simulink model "My_Nonlinear_with_controller_draft"  (R2021b)
settings: Solver=VariableStepAuto  StartTime=0.0  StopTime=simTime  RelTol=1e-3
undefined symbols (not defined in the file): att_Kd, att_Ki, att_Kp, b, D, g, k, L, m, MoI, omega, p, p_dot, posZ_Kd, posZ_Ki, posZ_Kp, posZ_N, Theta, TorV
libraries: slpidlib x8
settings Model: Creator=tanzc  LastModifiedBy=tanzc

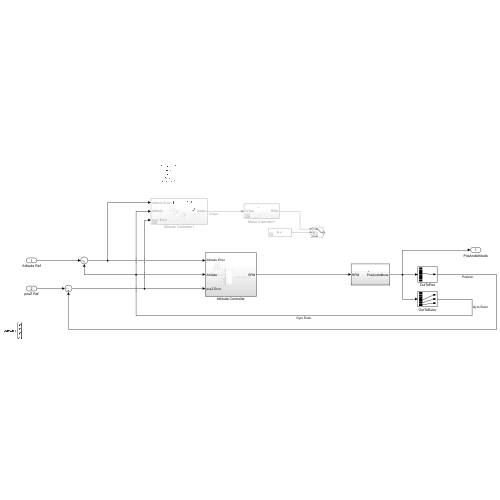
[thumbnail: Simulink's stored preview of the top-level diagram]
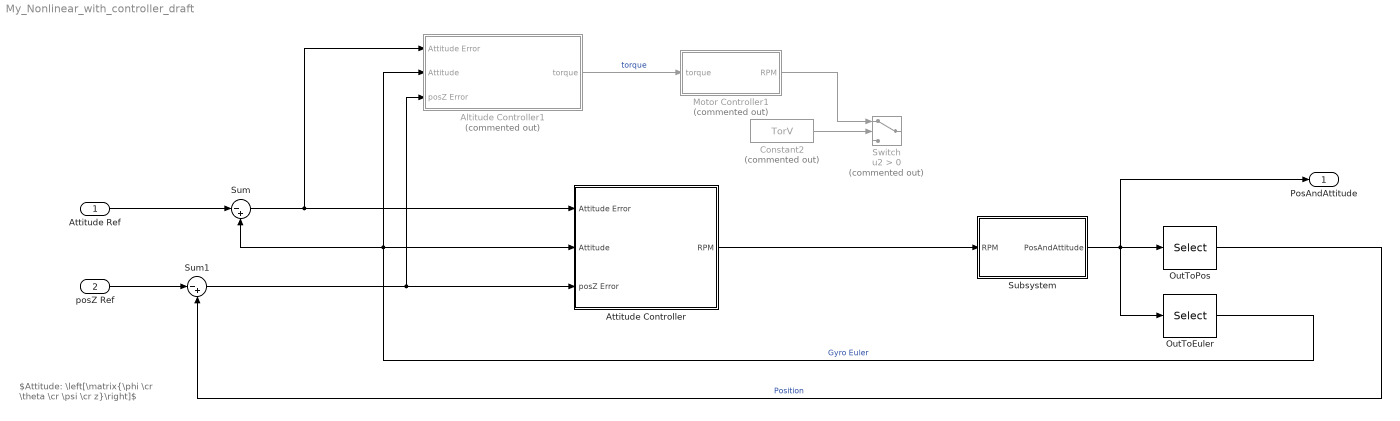
== system My_Nonlinear_with_controller_draft ==
  note: $Attitude: \left[\matrix{\phi \cr \theta \cr \psi \cr z}\right]$
  Attitude Ref : Inport  PortDimensions=3
  posZ Ref : Inport  Port=2  PortDimensions=1
  Altitude Controller1 : Subsystem  Commented=on
  Attitude Controller : Subsystem
  Constant2 : Constant  Commented=on  Value=TorV
  Motor Controller1 : Subsystem  Commented=on
  OutToEuler : Selector  InputPortWidth=6  IndexOptions=Index vector (dialog)  Indices=[4 5 6]  OutputSizes=1
  OutToPos : Selector  InputPortWidth=6  IndexOptions=Index vector (dialog)  Indices=[3]  OutputSizes=1
  Subsystem : Subsystem
  Sum : Sum  Inputs=|-+
  Sum1 : Sum  Inputs=|-+
  Switch : Switch  Commented=on  Criteria=u2 > Threshold
  PosAndAttitude : Outport
  wires:
  Subsystem/1(PosAndAttitude) -> PosAndAttitude/1, OutToEuler/1, OutToPos/1
  OutToPos/1 -> Sum1/2  "Position"
  OutToEuler/1 -> Altitude Controller1/2(Attitude), Attitude Controller/2(Attitude), Sum/2  "Gyro Euler"
  Sum/1 -> Altitude Controller1/1(Attitude Error), Attitude Controller/1(Attitude Error)
  Attitude Ref/1 -> Sum/1
  posZ Ref/1 -> Sum1/1
  Sum1/1 -> Altitude Controller1/3(posZ Error), Attitude Controller/3(posZ Error)
  Motor Controller1/1(RPM) -> Switch/1
  Constant2/1 -> Switch/2
  Altitude Controller1/1(torque) -> Motor Controller1/1(torque)  "torque"
  Attitude Controller/1(RPM) -> Subsystem/1(RPM)

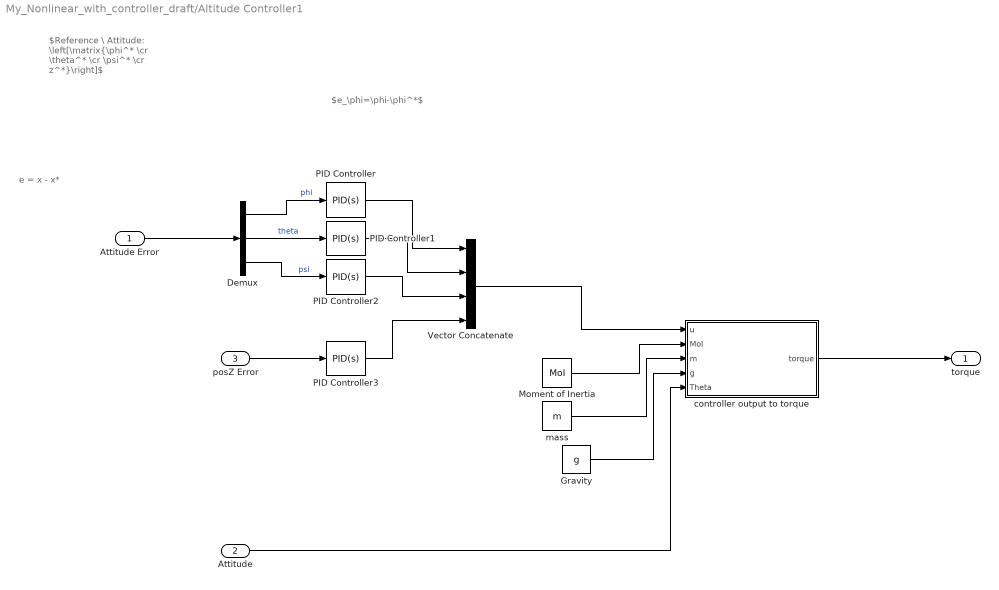
== system My_Nonlinear_with_controller_draft/Altitude Controller1 ==
  note: e = x - x*
  note: $e_\phi=\phi-\phi^*$
  note: $Reference \ Attitude: \left[\matrix{\phi^* \cr \theta^* \cr \psi^* \cr z^*}\right]$
  Attitude Error : Inport
  Attitude : Inport  Port=2
  posZ Error : Inport  Port=3
  Demux : Demux  Outputs=3
  Gravity : Constant  Value=g  VectorParams1D=off
  Moment of Inertia : Constant  Value=MoI  VectorParams1D=off
  PID Controller : slpidlib/PID Controller  Controller=PID  Form=Parallel  TimeDomain=Continuous-time  UseExternalTs=off  SampleTime=-1  IntegratorMethod=Forward Euler  FilterMethod=Forward Euler  ControllerParametersSource=internal  P=att_Kp  I=att_Ki  D=att_Kd  UseFilter=on  N=100  TunerSelectOption=Transfer Function Based (PID Tuner App)  InitialConditionSource=internal  InitialConditionForIntegrator=0  InitialConditionForFilter=0  DifferentiatorICPrevScaledInput=0  ExternalReset=none  TrackingMode=off  Kt=1  LimitOutput=off  SatLimitsSource=internal  UpperSaturationLimit=inf  LowerSaturationLimit=-inf  LinearizeAsGain=on  AntiWindupMode=none  Kb=1  POutMin=[]  POutMax=[]  IOutMin=[]  IOutMax=[]  DOutMin=[]  DOutMax=[]  NOutMin=[]  NOutMax=[]  SumOutMin=[]  SumOutMax=[]  SaturationOutMin=[]  SaturationOutMax=[]  PParamMin=[]  PParamMax=[]  IParamMin=[]  IParamMax=[]  DParamMin=[]  DParamMax=[]  NParamMin=[]  NParamMax=[]  KbParamMin=[]  KbParamMax=[]  KtParamMin=[]  KtParamMax=[]  KbOutMin=[]  KbOutMax=[]  KtOutMin=[]  KtOutMax=[]  IntegratorOutMin=[]  IntegratorOutMax=[]  FilterOutMin=[]  FilterOutMax=[]  SumI1OutMin=[]  SumI1OutMax=[]  SumI2OutMin=[]  SumI2OutMax=[]  SumI3OutMin=[]  SumI3OutMax=[]  SumI4OutMin=[]  SumI4OutMax=[]  SumDOutMin=[]  SumDOutMax=[]  DifferentiatorOutMin=[]  DifferentiatorOutMax=[]  FilterDiffOutCoefMin=[]  FilterDiffOutCoefMax=[]  ReciprocalOutMin=[]  ReciprocalOutMax=[]  SumDenOutMin=[]  SumDenOutMax=[]  SumNumOutMin=[]  SumNumOutMax=[]  DivideOutMin=[]  DivideOutMax=[]  UdiffTsProdOutMin=[]  UdiffTsProdOutMax=[]  NTsProdOutMin=[]  NTsProdOutMax=[]  UintegralTsProdOutMin=[]  UintegralTsProdOutMax=[]  UngainTsProdOutMin=[]  UngainTsProdOutMax=[]  IntegratorContinuousStateAttributes=''  IntegratorStateMustResolveToSignalObject=off  IntegratorRTWStateStorageClass=Auto  FilterContinuousStateAttributes=''  FilterStateMustResolveToSignalObject=off  FilterRTWStateStorageClass=Auto  ParallelPVariant=InternalParameters  IdealPVariant=Disabled  IVariant=InternalParameters  DVariant=InternalParameters  IntegratorVariant=Continuous  SatVariant=Disabled  AWVariant=Passthrough  PCopyVariant=Disabled  TRVariant=Disabled  FdbkBlocksVariant=Forward  IdealPFdbkVariant=Disabled  SatFdbkVariant=Disabled  DerivativeFilterVariant=ContFilter  NVariant=InternalParameters  NCopyVariant=Disabled  FilterICVariant=InternalICsFilter  IntegratorICVariant=InternalICs  ExternalResetVariant=Disabled  TRSumVariant=Passthrough  SumFdbkVariant=Disabled  SumVariant=Sum_PID  TsampFilterVariant=InternalTs  TsampNgainVariant=Passthrough  TsampIntegralVariant=Passthrough  ExternalSaturationOutDataTypeStr=Inherit: Same as second input
  PID Controller1 : slpidlib/PID Controller  Controller=PID  Form=Parallel  TimeDomain=Continuous-time  UseExternalTs=off  SampleTime=-1  IntegratorMethod=Forward Euler  FilterMethod=Forward Euler  ControllerParametersSource=internal  P=att_Kp  I=att_Ki  D=att_Kd  UseFilter=on  N=100  TunerSelectOption=Transfer Function Based (PID Tuner App)  InitialConditionSource=internal  InitialConditionForIntegrator=0  InitialConditionForFilter=0  DifferentiatorICPrevScaledInput=0  ExternalReset=none  TrackingMode=off  Kt=1  LimitOutput=off  SatLimitsSource=internal  UpperSaturationLimit=inf  LowerSaturationLimit=-inf  LinearizeAsGain=on  AntiWindupMode=none  Kb=1  POutMin=[]  POutMax=[]  IOutMin=[]  IOutMax=[]  DOutMin=[]  DOutMax=[]  NOutMin=[]  NOutMax=[]  SumOutMin=[]  SumOutMax=[]  SaturationOutMin=[]  SaturationOutMax=[]  PParamMin=[]  PParamMax=[]  IParamMin=[]  IParamMax=[]  DParamMin=[]  DParamMax=[]  NParamMin=[]  NParamMax=[]  KbParamMin=[]  KbParamMax=[]  KtParamMin=[]  KtParamMax=[]  KbOutMin=[]  KbOutMax=[]  KtOutMin=[]  KtOutMax=[]  IntegratorOutMin=[]  IntegratorOutMax=[]  FilterOutMin=[]  FilterOutMax=[]  SumI1OutMin=[]  SumI1OutMax=[]  SumI2OutMin=[]  SumI2OutMax=[]  SumI3OutMin=[]  SumI3OutMax=[]  SumI4OutMin=[]  SumI4OutMax=[]  SumDOutMin=[]  SumDOutMax=[]  DifferentiatorOutMin=[]  DifferentiatorOutMax=[]  FilterDiffOutCoefMin=[]  FilterDiffOutCoefMax=[]  ReciprocalOutMin=[]  ReciprocalOutMax=[]  SumDenOutMin=[]  SumDenOutMax=[]  SumNumOutMin=[]  SumNumOutMax=[]  DivideOutMin=[]  DivideOutMax=[]  UdiffTsProdOutMin=[]  UdiffTsProdOutMax=[]  NTsProdOutMin=[]  NTsProdOutMax=[]  UintegralTsProdOutMin=[]  UintegralTsProdOutMax=[]  UngainTsProdOutMin=[]  UngainTsProdOutMax=[]  IntegratorContinuousStateAttributes=''  IntegratorStateMustResolveToSignalObject=off  IntegratorRTWStateStorageClass=Auto  FilterContinuousStateAttributes=''  FilterStateMustResolveToSignalObject=off  FilterRTWStateStorageClass=Auto  ParallelPVariant=InternalParameters  IdealPVariant=Disabled  IVariant=InternalParameters  DVariant=InternalParameters  IntegratorVariant=Continuous  SatVariant=Disabled  AWVariant=Passthrough  PCopyVariant=Disabled  TRVariant=Disabled  FdbkBlocksVariant=Forward  IdealPFdbkVariant=Disabled  SatFdbkVariant=Disabled  DerivativeFilterVariant=ContFilter  NVariant=InternalParameters  NCopyVariant=Disabled  FilterICVariant=InternalICsFilter  IntegratorICVariant=InternalICs  ExternalResetVariant=Disabled  TRSumVariant=Passthrough  SumFdbkVariant=Disabled  SumVariant=Sum_PID  TsampFilterVariant=InternalTs  TsampNgainVariant=Passthrough  TsampIntegralVariant=Passthrough  ExternalSaturationOutDataTypeStr=Inherit: Same as second input
  PID Controller2 : slpidlib/PID Controller  Controller=PID  Form=Parallel  TimeDomain=Continuous-time  UseExternalTs=off  SampleTime=-1  IntegratorMethod=Forward Euler  FilterMethod=Forward Euler  ControllerParametersSource=internal  P=att_Kp  I=att_Ki  D=att_Kd  UseFilter=on  N=100  TunerSelectOption=Transfer Function Based (PID Tuner App)  InitialConditionSource=internal  InitialConditionForIntegrator=0  InitialConditionForFilter=0  DifferentiatorICPrevScaledInput=0  ExternalReset=none  TrackingMode=off  Kt=1  LimitOutput=off  SatLimitsSource=internal  UpperSaturationLimit=inf  LowerSaturationLimit=-inf  LinearizeAsGain=on  AntiWindupMode=none  Kb=1  POutMin=[]  POutMax=[]  IOutMin=[]  IOutMax=[]  DOutMin=[]  DOutMax=[]  NOutMin=[]  NOutMax=[]  SumOutMin=[]  SumOutMax=[]  SaturationOutMin=[]  SaturationOutMax=[]  PParamMin=[]  PParamMax=[]  IParamMin=[]  IParamMax=[]  DParamMin=[]  DParamMax=[]  NParamMin=[]  NParamMax=[]  KbParamMin=[]  KbParamMax=[]  KtParamMin=[]  KtParamMax=[]  KbOutMin=[]  KbOutMax=[]  KtOutMin=[]  KtOutMax=[]  IntegratorOutMin=[]  IntegratorOutMax=[]  FilterOutMin=[]  FilterOutMax=[]  SumI1OutMin=[]  SumI1OutMax=[]  SumI2OutMin=[]  SumI2OutMax=[]  SumI3OutMin=[]  SumI3OutMax=[]  SumI4OutMin=[]  SumI4OutMax=[]  SumDOutMin=[]  SumDOutMax=[]  DifferentiatorOutMin=[]  DifferentiatorOutMax=[]  FilterDiffOutCoefMin=[]  FilterDiffOutCoefMax=[]  ReciprocalOutMin=[]  ReciprocalOutMax=[]  SumDenOutMin=[]  SumDenOutMax=[]  SumNumOutMin=[]  SumNumOutMax=[]  DivideOutMin=[]  DivideOutMax=[]  UdiffTsProdOutMin=[]  UdiffTsProdOutMax=[]  NTsProdOutMin=[]  NTsProdOutMax=[]  UintegralTsProdOutMin=[]  UintegralTsProdOutMax=[]  UngainTsProdOutMin=[]  UngainTsProdOutMax=[]  IntegratorContinuousStateAttributes=''  IntegratorStateMustResolveToSignalObject=off  IntegratorRTWStateStorageClass=Auto  FilterContinuousStateAttributes=''  FilterStateMustResolveToSignalObject=off  FilterRTWStateStorageClass=Auto  ParallelPVariant=InternalParameters  IdealPVariant=Disabled  IVariant=InternalParameters  DVariant=InternalParameters  IntegratorVariant=Continuous  SatVariant=Disabled  AWVariant=Passthrough  PCopyVariant=Disabled  TRVariant=Disabled  FdbkBlocksVariant=Forward  IdealPFdbkVariant=Disabled  SatFdbkVariant=Disabled  DerivativeFilterVariant=ContFilter  NVariant=InternalParameters  NCopyVariant=Disabled  FilterICVariant=InternalICsFilter  IntegratorICVariant=InternalICs  ExternalResetVariant=Disabled  TRSumVariant=Passthrough  SumFdbkVariant=Disabled  SumVariant=Sum_PID  TsampFilterVariant=InternalTs  TsampNgainVariant=Passthrough  TsampIntegralVariant=Passthrough  ExternalSaturationOutDataTypeStr=Inherit: Same as second input
  PID Controller3 : slpidlib/PID Controller  Controller=PID  Form=Parallel  TimeDomain=Continuous-time  UseExternalTs=off  SampleTime=-1  IntegratorMethod=Forward Euler  FilterMethod=Forward Euler  ControllerParametersSource=internal  P=posZ_Kp  I=posZ_Ki  D=posZ_Kd  UseFilter=on  N=100  TunerSelectOption=Transfer Function Based (PID Tuner App)  InitialConditionSource=internal  InitialConditionForIntegrator=0  InitialConditionForFilter=0  DifferentiatorICPrevScaledInput=0  ExternalReset=none  TrackingMode=off  Kt=1  LimitOutput=off  SatLimitsSource=internal  UpperSaturationLimit=inf  LowerSaturationLimit=-inf  LinearizeAsGain=on  AntiWindupMode=none  Kb=1  POutMin=[]  POutMax=[]  IOutMin=[]  IOutMax=[]  DOutMin=[]  DOutMax=[]  NOutMin=[]  NOutMax=[]  SumOutMin=[]  SumOutMax=[]  SaturationOutMin=[]  SaturationOutMax=[]  PParamMin=[]  PParamMax=[]  IParamMin=[]  IParamMax=[]  DParamMin=[]  DParamMax=[]  NParamMin=[]  NParamMax=[]  KbParamMin=[]  KbParamMax=[]  KtParamMin=[]  KtParamMax=[]  KbOutMin=[]  KbOutMax=[]  KtOutMin=[]  KtOutMax=[]  IntegratorOutMin=[]  IntegratorOutMax=[]  FilterOutMin=[]  FilterOutMax=[]  SumI1OutMin=[]  SumI1OutMax=[]  SumI2OutMin=[]  SumI2OutMax=[]  SumI3OutMin=[]  SumI3OutMax=[]  SumI4OutMin=[]  SumI4OutMax=[]  SumDOutMin=[]  SumDOutMax=[]  DifferentiatorOutMin=[]  DifferentiatorOutMax=[]  FilterDiffOutCoefMin=[]  FilterDiffOutCoefMax=[]  ReciprocalOutMin=[]  ReciprocalOutMax=[]  SumDenOutMin=[]  SumDenOutMax=[]  SumNumOutMin=[]  SumNumOutMax=[]  DivideOutMin=[]  DivideOutMax=[]  UdiffTsProdOutMin=[]  UdiffTsProdOutMax=[]  NTsProdOutMin=[]  NTsProdOutMax=[]  UintegralTsProdOutMin=[]  UintegralTsProdOutMax=[]  UngainTsProdOutMin=[]  UngainTsProdOutMax=[]  IntegratorContinuousStateAttributes=''  IntegratorStateMustResolveToSignalObject=off  IntegratorRTWStateStorageClass=Auto  FilterContinuousStateAttributes=''  FilterStateMustResolveToSignalObject=off  FilterRTWStateStorageClass=Auto  ParallelPVariant=InternalParameters  IdealPVariant=Disabled  IVariant=InternalParameters  DVariant=InternalParameters  IntegratorVariant=Continuous  SatVariant=Disabled  AWVariant=Passthrough  PCopyVariant=Disabled  TRVariant=Disabled  FdbkBlocksVariant=Forward  IdealPFdbkVariant=Disabled  SatFdbkVariant=Disabled  DerivativeFilterVariant=ContFilter  NVariant=InternalParameters  NCopyVariant=Disabled  FilterICVariant=InternalICsFilter  IntegratorICVariant=InternalICs  ExternalResetVariant=Disabled  TRSumVariant=Passthrough  SumFdbkVariant=Disabled  SumVariant=Sum_PID  TsampFilterVariant=InternalTs  TsampNgainVariant=Passthrough  TsampIntegralVariant=Passthrough  ExternalSaturationOutDataTypeStr=Inherit: Same as second input
  Vector Concatenate : Concatenate  NumInputs=4
  controller output to torque : MATLAB Function  TreatAsAtomicUnit=on
  mass : Constant  Value=m
  torque : Outport
  wires:
  Attitude Error/1 -> Demux/1
  Attitude/1 -> controller output to torque/5(Theta)
  Vector Concatenate/1 -> controller output to torque/1(u)
  Moment of Inertia/1 -> controller output to torque/2(MoI)
  mass/1 -> controller output to torque/3(m)
  Gravity/1 -> controller output to torque/4(g)
  controller output to torque/1(torque) -> torque/1
  Demux/1 -> PID Controller/1  "phi"
  Demux/2 -> PID Controller1/1  "theta"
  Demux/3 -> PID Controller2/1  "psi"
  posZ Error/1 -> PID Controller3/1
  PID Controller/1 -> Vector Concatenate/1
  PID Controller1/1 -> Vector Concatenate/2
  PID Controller2/1 -> Vector Concatenate/3
  PID Controller3/1 -> Vector Concatenate/4

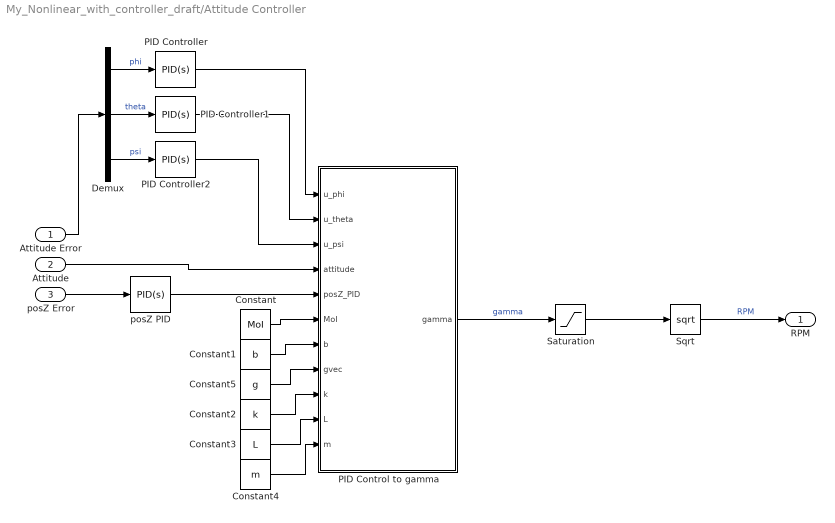
== system My_Nonlinear_with_controller_draft/Attitude Controller ==
  Attitude Error : Inport  PortDimensions=3
  Attitude : Inport  Port=2  PortDimensions=3
  posZ Error : Inport  Port=3
  Constant : Constant  Value=MoI
  Constant1 : Constant  Value=b
  Constant2 : Constant  Value=k
  Constant3 : Constant  Value=L
  Constant4 : Constant  Value=m
  Constant5 : Constant  Value=g
  Demux : Demux  Outputs=3
  PID Control to gamma : MATLAB Function  TreatAsAtomicUnit=on
  PID Controller : slpidlib/PID Controller  Priority=1  Controller=PID  Form=Parallel  TimeDomain=Continuous-time  UseExternalTs=off  SampleTime=-1  IntegratorMethod=Forward Euler  FilterMethod=Forward Euler  ControllerParametersSource=internal  P=att_Kp  I=att_Ki  D=att_Kd  UseFilter=on  N=1142.8279760416  TunerSelectOption=Transfer Function Based (PID Tuner App)  InitialConditionSource=internal  InitialConditionForIntegrator=0  InitialConditionForFilter=0  DifferentiatorICPrevScaledInput=0  ExternalReset=none  TrackingMode=off  Kt=1  LimitOutput=off  SatLimitsSource=internal  UpperSaturationLimit=inf  LowerSaturationLimit=-inf  LinearizeAsGain=on  AntiWindupMode=none  Kb=1  POutMin=[]  POutMax=[]  IOutMin=[]  IOutMax=[]  DOutMin=[]  DOutMax=[]  NOutMin=[]  NOutMax=[]  SumOutMin=[]  SumOutMax=[]  SaturationOutMin=[]  SaturationOutMax=[]  PParamMin=[]  PParamMax=[]  IParamMin=[]  IParamMax=[]  DParamMin=[]  DParamMax=[]  NParamMin=[]  NParamMax=[]  KbParamMin=[]  KbParamMax=[]  KtParamMin=[]  KtParamMax=[]  KbOutMin=[]  KbOutMax=[]  KtOutMin=[]  KtOutMax=[]  IntegratorOutMin=[]  IntegratorOutMax=[]  FilterOutMin=[]  FilterOutMax=[]  SumI1OutMin=[]  SumI1OutMax=[]  SumI2OutMin=[]  SumI2OutMax=[]  SumI3OutMin=[]  SumI3OutMax=[]  SumI4OutMin=[]  SumI4OutMax=[]  SumDOutMin=[]  SumDOutMax=[]  DifferentiatorOutMin=[]  DifferentiatorOutMax=[]  FilterDiffOutCoefMin=[]  FilterDiffOutCoefMax=[]  ReciprocalOutMin=[]  ReciprocalOutMax=[]  SumDenOutMin=[]  SumDenOutMax=[]  SumNumOutMin=[]  SumNumOutMax=[]  DivideOutMin=[]  DivideOutMax=[]  UdiffTsProdOutMin=[]  UdiffTsProdOutMax=[]  NTsProdOutMin=[]  NTsProdOutMax=[]  UintegralTsProdOutMin=[]  UintegralTsProdOutMax=[]  UngainTsProdOutMin=[]  UngainTsProdOutMax=[]  IntegratorContinuousStateAttributes=''  IntegratorStateMustResolveToSignalObject=off  IntegratorRTWStateStorageClass=Auto  FilterContinuousStateAttributes=''  FilterStateMustResolveToSignalObject=off  FilterRTWStateStorageClass=Auto  ParallelPVariant=InternalParameters  IdealPVariant=Disabled  IVariant=InternalParameters  DVariant=InternalParameters  IntegratorVariant=Continuous  SatVariant=Disabled  AWVariant=Passthrough  PCopyVariant=Disabled  TRVariant=Disabled  FdbkBlocksVariant=Forward  IdealPFdbkVariant=Disabled  SatFdbkVariant=Disabled  DerivativeFilterVariant=ContFilter  NVariant=InternalParameters  NCopyVariant=Disabled  FilterICVariant=InternalICsFilter  IntegratorICVariant=InternalICs  ExternalResetVariant=Disabled  TRSumVariant=Passthrough  SumFdbkVariant=Disabled  SumVariant=Sum_PID  TsampFilterVariant=InternalTs  TsampNgainVariant=Passthrough  TsampIntegralVariant=Passthrough  ExternalSaturationOutDataTypeStr=Inherit: Same as second input
  PID Controller1 : slpidlib/PID Controller  Priority=2  Controller=PID  Form=Parallel  TimeDomain=Continuous-time  UseExternalTs=off  SampleTime=-1  IntegratorMethod=Forward Euler  FilterMethod=Forward Euler  ControllerParametersSource=internal  P=att_Kp  I=att_Ki  D=att_Kd  UseFilter=on  N=100  TunerSelectOption=Transfer Function Based (PID Tuner App)  InitialConditionSource=internal  InitialConditionForIntegrator=0  InitialConditionForFilter=0  DifferentiatorICPrevScaledInput=0  ExternalReset=none  TrackingMode=off  Kt=1  LimitOutput=off  SatLimitsSource=internal  UpperSaturationLimit=inf  LowerSaturationLimit=-inf  LinearizeAsGain=on  AntiWindupMode=none  Kb=1  POutMin=[]  POutMax=[]  IOutMin=[]  IOutMax=[]  DOutMin=[]  DOutMax=[]  NOutMin=[]  NOutMax=[]  SumOutMin=[]  SumOutMax=[]  SaturationOutMin=[]  SaturationOutMax=[]  PParamMin=[]  PParamMax=[]  IParamMin=[]  IParamMax=[]  DParamMin=[]  DParamMax=[]  NParamMin=[]  NParamMax=[]  KbParamMin=[]  KbParamMax=[]  KtParamMin=[]  KtParamMax=[]  KbOutMin=[]  KbOutMax=[]  KtOutMin=[]  KtOutMax=[]  IntegratorOutMin=[]  IntegratorOutMax=[]  FilterOutMin=[]  FilterOutMax=[]  SumI1OutMin=[]  SumI1OutMax=[]  SumI2OutMin=[]  SumI2OutMax=[]  SumI3OutMin=[]  SumI3OutMax=[]  SumI4OutMin=[]  SumI4OutMax=[]  SumDOutMin=[]  SumDOutMax=[]  DifferentiatorOutMin=[]  DifferentiatorOutMax=[]  FilterDiffOutCoefMin=[]  FilterDiffOutCoefMax=[]  ReciprocalOutMin=[]  ReciprocalOutMax=[]  SumDenOutMin=[]  SumDenOutMax=[]  SumNumOutMin=[]  SumNumOutMax=[]  DivideOutMin=[]  DivideOutMax=[]  UdiffTsProdOutMin=[]  UdiffTsProdOutMax=[]  NTsProdOutMin=[]  NTsProdOutMax=[]  UintegralTsProdOutMin=[]  UintegralTsProdOutMax=[]  UngainTsProdOutMin=[]  UngainTsProdOutMax=[]  IntegratorContinuousStateAttributes=''  IntegratorStateMustResolveToSignalObject=off  IntegratorRTWStateStorageClass=Auto  FilterContinuousStateAttributes=''  FilterStateMustResolveToSignalObject=off  FilterRTWStateStorageClass=Auto  ParallelPVariant=InternalParameters  IdealPVariant=Disabled  IVariant=InternalParameters  DVariant=InternalParameters  IntegratorVariant=Continuous  SatVariant=Disabled  AWVariant=Passthrough  PCopyVariant=Disabled  TRVariant=Disabled  FdbkBlocksVariant=Forward  IdealPFdbkVariant=Disabled  SatFdbkVariant=Disabled  DerivativeFilterVariant=ContFilter  NVariant=InternalParameters  NCopyVariant=Disabled  FilterICVariant=InternalICsFilter  IntegratorICVariant=InternalICs  ExternalResetVariant=Disabled  TRSumVariant=Passthrough  SumFdbkVariant=Disabled  SumVariant=Sum_PID  TsampFilterVariant=InternalTs  TsampNgainVariant=Passthrough  TsampIntegralVariant=Passthrough  ExternalSaturationOutDataTypeStr=Inherit: Same as second input
  PID Controller2 : slpidlib/PID Controller  Priority=3  Controller=PID  Form=Parallel  TimeDomain=Continuous-time  UseExternalTs=off  SampleTime=-1  IntegratorMethod=Forward Euler  FilterMethod=Forward Euler  ControllerParametersSource=internal  P=att_Kp  I=att_Ki  D=att_Kd  UseFilter=on  N=100  TunerSelectOption=Transfer Function Based (PID Tuner App)  InitialConditionSource=internal  InitialConditionForIntegrator=0  InitialConditionForFilter=0  DifferentiatorICPrevScaledInput=0  ExternalReset=none  TrackingMode=off  Kt=1  LimitOutput=off  SatLimitsSource=internal  UpperSaturationLimit=inf  LowerSaturationLimit=-inf  LinearizeAsGain=on  AntiWindupMode=none  Kb=1  POutMin=[]  POutMax=[]  IOutMin=[]  IOutMax=[]  DOutMin=[]  DOutMax=[]  NOutMin=[]  NOutMax=[]  SumOutMin=[]  SumOutMax=[]  SaturationOutMin=[]  SaturationOutMax=[]  PParamMin=[]  PParamMax=[]  IParamMin=[]  IParamMax=[]  DParamMin=[]  DParamMax=[]  NParamMin=[]  NParamMax=[]  KbParamMin=[]  KbParamMax=[]  KtParamMin=[]  KtParamMax=[]  KbOutMin=[]  KbOutMax=[]  KtOutMin=[]  KtOutMax=[]  IntegratorOutMin=[]  IntegratorOutMax=[]  FilterOutMin=[]  FilterOutMax=[]  SumI1OutMin=[]  SumI1OutMax=[]  SumI2OutMin=[]  SumI2OutMax=[]  SumI3OutMin=[]  SumI3OutMax=[]  SumI4OutMin=[]  SumI4OutMax=[]  SumDOutMin=[]  SumDOutMax=[]  DifferentiatorOutMin=[]  DifferentiatorOutMax=[]  FilterDiffOutCoefMin=[]  FilterDiffOutCoefMax=[]  ReciprocalOutMin=[]  ReciprocalOutMax=[]  SumDenOutMin=[]  SumDenOutMax=[]  SumNumOutMin=[]  SumNumOutMax=[]  DivideOutMin=[]  DivideOutMax=[]  UdiffTsProdOutMin=[]  UdiffTsProdOutMax=[]  NTsProdOutMin=[]  NTsProdOutMax=[]  UintegralTsProdOutMin=[]  UintegralTsProdOutMax=[]  UngainTsProdOutMin=[]  UngainTsProdOutMax=[]  IntegratorContinuousStateAttributes=''  IntegratorStateMustResolveToSignalObject=off  IntegratorRTWStateStorageClass=Auto  FilterContinuousStateAttributes=''  FilterStateMustResolveToSignalObject=off  FilterRTWStateStorageClass=Auto  ParallelPVariant=InternalParameters  IdealPVariant=Disabled  IVariant=InternalParameters  DVariant=InternalParameters  IntegratorVariant=Continuous  SatVariant=Disabled  AWVariant=Passthrough  PCopyVariant=Disabled  TRVariant=Disabled  FdbkBlocksVariant=Forward  IdealPFdbkVariant=Disabled  SatFdbkVariant=Disabled  DerivativeFilterVariant=ContFilter  NVariant=InternalParameters  NCopyVariant=Disabled  FilterICVariant=InternalICsFilter  IntegratorICVariant=InternalICs  ExternalResetVariant=Disabled  TRSumVariant=Passthrough  SumFdbkVariant=Disabled  SumVariant=Sum_PID  TsampFilterVariant=InternalTs  TsampNgainVariant=Passthrough  TsampIntegralVariant=Passthrough  ExternalSaturationOutDataTypeStr=Inherit: Same as second input
  Saturation : Saturate  UpperLimit=100000  LowerLimit=0
  Sqrt : Sqrt  SaturateOnIntegerOverflow=on
  posZ PID : slpidlib/PID Controller  Priority=4  Controller=PID  Form=Parallel  TimeDomain=Continuous-time  UseExternalTs=off  SampleTime=-1  IntegratorMethod=Forward Euler  FilterMethod=Forward Euler  ControllerParametersSource=internal  P=posZ_Kp  I=posZ_Ki  D=posZ_Kd  UseFilter=on  N=posZ_N  TunerSelectOption=Transfer Function Based (PID Tuner App)  InitialConditionSource=internal  InitialConditionForIntegrator=0  InitialConditionForFilter=0  DifferentiatorICPrevScaledInput=0  ExternalReset=none  TrackingMode=off  Kt=1  LimitOutput=off  SatLimitsSource=internal  UpperSaturationLimit=inf  LowerSaturationLimit=-inf  LinearizeAsGain=on  AntiWindupMode=none  Kb=1  POutMin=[]  POutMax=[]  IOutMin=[]  IOutMax=[]  DOutMin=[]  DOutMax=[]  NOutMin=[]  NOutMax=[]  SumOutMin=[]  SumOutMax=[]  SaturationOutMin=[]  SaturationOutMax=[]  PParamMin=[]  PParamMax=[]  IParamMin=[]  IParamMax=[]  DParamMin=[]  DParamMax=[]  NParamMin=[]  NParamMax=[]  KbParamMin=[]  KbParamMax=[]  KtParamMin=[]  KtParamMax=[]  KbOutMin=[]  KbOutMax=[]  KtOutMin=[]  KtOutMax=[]  IntegratorOutMin=[]  IntegratorOutMax=[]  FilterOutMin=[]  FilterOutMax=[]  SumI1OutMin=[]  SumI1OutMax=[]  SumI2OutMin=[]  SumI2OutMax=[]  SumI3OutMin=[]  SumI3OutMax=[]  SumI4OutMin=[]  SumI4OutMax=[]  SumDOutMin=[]  SumDOutMax=[]  DifferentiatorOutMin=[]  DifferentiatorOutMax=[]  FilterDiffOutCoefMin=[]  FilterDiffOutCoefMax=[]  ReciprocalOutMin=[]  ReciprocalOutMax=[]  SumDenOutMin=[]  SumDenOutMax=[]  SumNumOutMin=[]  SumNumOutMax=[]  DivideOutMin=[]  DivideOutMax=[]  UdiffTsProdOutMin=[]  UdiffTsProdOutMax=[]  NTsProdOutMin=[]  NTsProdOutMax=[]  UintegralTsProdOutMin=[]  UintegralTsProdOutMax=[]  UngainTsProdOutMin=[]  UngainTsProdOutMax=[]  IntegratorContinuousStateAttributes=''  IntegratorStateMustResolveToSignalObject=off  IntegratorRTWStateStorageClass=Auto  FilterContinuousStateAttributes=''  FilterStateMustResolveToSignalObject=off  FilterRTWStateStorageClass=Auto  ParallelPVariant=InternalParameters  IdealPVariant=Disabled  IVariant=InternalParameters  DVariant=InternalParameters  IntegratorVariant=Continuous  SatVariant=Disabled  AWVariant=Passthrough  PCopyVariant=Disabled  TRVariant=Disabled  FdbkBlocksVariant=Forward  IdealPFdbkVariant=Disabled  SatFdbkVariant=Disabled  DerivativeFilterVariant=ContFilter  NVariant=InternalParameters  NCopyVariant=Disabled  FilterICVariant=InternalICsFilter  IntegratorICVariant=InternalICs  ExternalResetVariant=Disabled  TRSumVariant=Passthrough  SumFdbkVariant=Disabled  SumVariant=Sum_PID  TsampFilterVariant=InternalTs  TsampNgainVariant=Passthrough  TsampIntegralVariant=Passthrough  ExternalSaturationOutDataTypeStr=Inherit: Same as second input
  RPM : Outport
  wires:
  Constant/1 -> PID Control to gamma/6(MoI)
  Constant1/1 -> PID Control to gamma/7(b)
  Constant2/1 -> PID Control to gamma/9(k)
  Constant3/1 -> PID Control to gamma/10(L)
  Constant4/1 -> PID Control to gamma/11(m)
  Constant5/1 -> PID Control to gamma/8(gvec)
  PID Control to gamma/1(gamma) -> Saturation/1  "gamma"
  Sqrt/1 -> RPM/1  "RPM"
  Attitude Error/1 -> Demux/1
  posZ Error/1 -> posZ PID/1
  posZ PID/1 -> PID Control to gamma/5(posZ_PID)
  Demux/1 -> PID Controller/1  "phi"
  Demux/2 -> PID Controller1/1  "theta"
  Demux/3 -> PID Controller2/1  "psi"
  Attitude/1 -> PID Control to gamma/4(attitude)
  PID Controller2/1 -> PID Control to gamma/3(u_psi)
  PID Controller1/1 -> PID Control to gamma/2(u_theta)
  PID Controller/1 -> PID Control to gamma/1(u_phi)
  Saturation/1 -> Sqrt/1

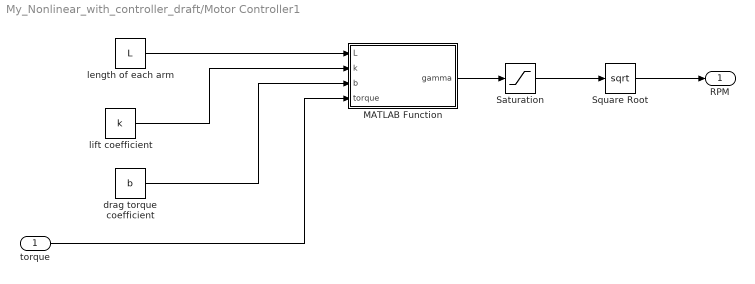
== system My_Nonlinear_with_controller_draft/Motor Controller1 ==
  torque : Inport
  MATLAB Function : MATLAB Function  TreatAsAtomicUnit=on
  Saturation : Saturate  UpperLimit=100000  LowerLimit=0
  Square Root : Sqrt  SaturateOnIntegerOverflow=on
  drag torque coefficient : Constant  Value=b
  length of each arm : Constant  Value=L
  lift coefficient : Constant  Value=k
  RPM : Outport
  wires:
  length of each arm/1 -> MATLAB Function/1(L)
  lift coefficient/1 -> MATLAB Function/2(k)
  drag torque coefficient/1 -> MATLAB Function/3(b)
  torque/1 -> MATLAB Function/4(torque)
  Square Root/1 -> RPM/1
  Saturation/1 -> Square Root/1
  MATLAB Function/1(gamma) -> Saturation/1

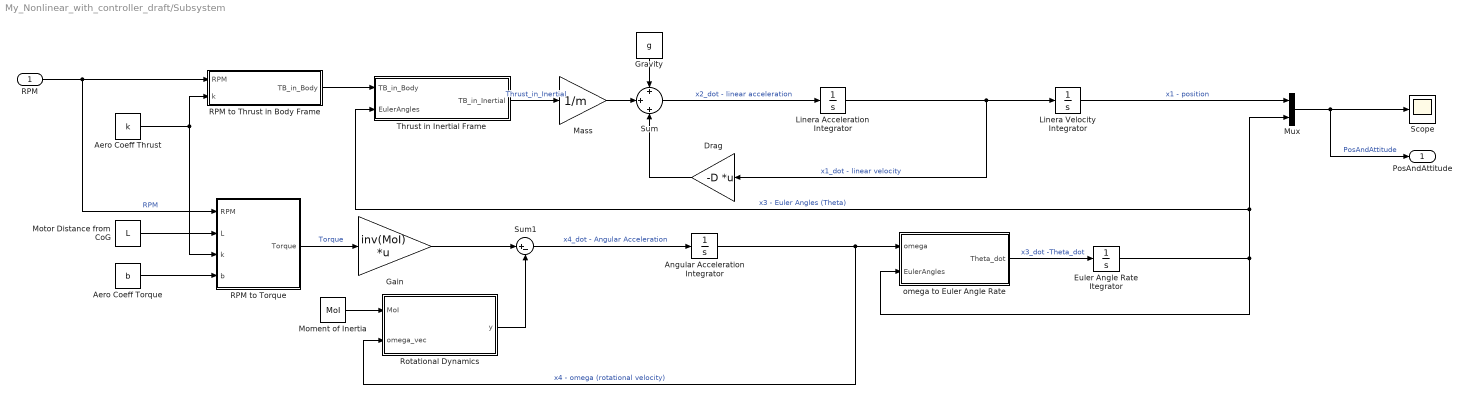
== system My_Nonlinear_with_controller_draft/Subsystem ==
  RPM : Inport
  Aero Coeff Thrust : Constant  Value=k
  Aero Coeff Torque : Constant  Value=b
  Angular Acceleration Integrator : Integrator  Priority=4  InitialCondition=omega
  Drag : Gain  Gain=-D  Multiplication=Matrix(K*u)
  Euler Angle Rate Itegrator : Integrator  Priority=3  InitialCondition=Theta
  Gain : Gain  Gain=inv(MoI)  Multiplication=Matrix(K*u)
  Gravity : Constant  Value=g  VectorParams1D=off
  Linera Acceleration Integrator : Integrator  Priority=2  InitialCondition=p_dot
  Linera Velocity Integrator : Integrator  Priority=1  InitialCondition=p
  Mass : Gain  Gain=1/m
  Moment of Inertia : Constant  Value=MoI  VectorParams1D=off
  Motor Distance from CoG : Constant  Value=L
  Mux : Mux  Inputs=2
  RPM to Thrust in Body Frame : MATLAB Function  TreatAsAtomicUnit=on
  RPM to Torque : MATLAB Function  TreatAsAtomicUnit=on
  Rotational Dynamics : MATLAB Function  TreatAsAtomicUnit=on
  Scope : Scope
  Sum : Sum  Inputs=+|+|+
  Sum1 : Sum  Inputs=|+-
  Thrust in Inertial Frame : MATLAB Function  TreatAsAtomicUnit=on
  "omega to Euler Angle Rate " : MATLAB Function  TreatAsAtomicUnit=on
  PosAndAttitude : Outport
  wires:
  Sum1/1 -> Angular Acceleration Integrator/1  "x4_dot - Angular Acceleration"
  Moment of Inertia/1 -> Rotational Dynamics/1(MoI)
  Mux/1 -> PosAndAttitude/1, Scope/1  "PosAndAttitude"
  Aero Coeff Torque/1 -> RPM to Torque/4(b)
  RPM/1 -> RPM to Thrust in Body Frame/1(RPM), RPM to Torque/1(RPM)  "RPM"
  Angular Acceleration Integrator/1 -> "omega to Euler Angle Rate "/1(omega), Rotational Dynamics/2(omega_vec)  "x4 - omega (rotational velocity)"
  Gain/1 -> Sum1/1
  RPM to Thrust in Body Frame/1(TB_in_Body) -> Thrust in Inertial Frame/1(TB_in_Body)
  Thrust in Inertial Frame/1(TB_in_Inertial) -> Mass/1  "Thrust_in_Inertial"
  Sum/1 -> Linera Acceleration Integrator/1  "x2_dot - linear acceleration"
  Rotational Dynamics/1(y) -> Sum1/2
  Drag/1 -> Sum/3
  Mass/1 -> Sum/2
  Gravity/1 -> Sum/1
  Motor Distance from CoG/1 -> RPM to Torque/2(L)
  RPM to Torque/1(Torque) -> Gain/1  "Torque"
  Linera Acceleration Integrator/1 -> Drag/1, Linera Velocity Integrator/1  "x1_dot - linear velocity"
  Aero Coeff Thrust/1 -> RPM to Thrust in Body Frame/2(k), RPM to Torque/3(k)
  Euler Angle Rate Itegrator/1 -> Thrust in Inertial Frame/2(EulerAngles), Mux/2, "omega to Euler Angle Rate "/2(EulerAngles)  "x3 - Euler Angles (Theta)"
  "omega to Euler Angle Rate "/1(Theta_dot) -> Euler Angle Rate Itegrator/1  "x3_dot -Theta_dot"
  Linera Velocity Integrator/1 -> Mux/1  "x1 - position"

== matlab function My_Nonlinear_with_controller_draft/Subsystem/RPM to Thrust in Body Frame ==
  data: RPM input; TB_in_Body output; k input
function TB_in_Body = fcn(RPM, k)
TB_in_Body = k * [0; 0; RPM'*RPM];

== matlab function My_Nonlinear_with_controller_draft/Subsystem/Thrust in Inertial Frame ==
  data: TB_in_Body input; EulerAngles input; TB_in_Inertial output
function TB_in_Inertial = fcn(TB_in_Body, EulerAngles)

phi = EulerAngles(1);
theta = EulerAngles(2);
psi = EulerAngles(3);

R = [cos(psi)*cos(theta), cos(psi)*sin(theta)*sin(phi) - sin(psi)*cos(phi), cos(psi)*sin(theta)*cos(phi) + sin(psi)*sin(phi);
    sin(psi)*cos(theta), sin(psi)*sin(theta)*sin(phi) + cos(psi)*cos(phi), sin(psi)*sin(theta)*cos(phi) - cos(psi)*sin(phi);
    -sin(theta), cos(theta)*sin(phi), cos(theta)*cos(phi)];

TB_in_Inertial = R*TB_in_Body;

== matlab function My_Nonlinear_with_controller_draft/Subsystem/RPM to Torque ==
  data: RPM input; Torque output; L input; k input; b input
function Torque = fcn(RPM, L, k, b)

Torque = [  L*k*(RPM(1)^2 - RPM(3)^2); ...
            L*k*(RPM(2)^2 - RPM(4)^2); ...
            b * (RPM(1)^2 - RPM(2)^2 + RPM(3)^2 - RPM(4)^2)];

== matlab function My_Nonlinear_with_controller_draft/Subsystem/Rotational Dynamics ==
  data: MoI input; omega_vec input; y output
function y = fcn(MoI, omega_vec)
Ixx = MoI(1,1);
Iyy = MoI(2,2);
Izz = MoI(3,3);

omega_x = omega_vec(1);
omega_y = omega_vec(2);
omega_z = omega_vec(3);

y = [ (Iyy-Izz)/Ixx*omega_y*omega_z; ...
      (Izz-Ixx)/Iyy*omega_x*omega_z; ...
      (Ixx-Iyy)/Izz*omega_x*omega_y];

== matlab function My_Nonlinear_with_controller_draft/Subsystem/omega to Euler Angle Rate  ==
  data: omega input; Theta_dot output; EulerAngles input
function Theta_dot = fcn(omega, EulerAngles)

phi = EulerAngles(1);
theta = EulerAngles(2);
psi = EulerAngles(3);

B = [ 1, 0, -sin(theta); ...
      0, cos(phi), cos(theta)*sin(phi); ...
      0, -sin(phi), cos(theta)*cos(phi)];
  
Theta_dot = pinv(B)*omega;

== matlab function My_Nonlinear_with_controller_draft/Attitude Controller/PID Control to gamma ==
  data: u_phi input; u_theta input; u_psi input; attitude input; gamma output; posZ_PID input; MoI input; b input; gvec input; k input; L input; m input
function gamma = fcn(u_phi, u_theta, u_psi, attitude, posZ_PID, MoI, b, gvec, k, L, m)

%u_phi   = att_PID(1);
%u_theta = att_PID(2);
%u_psi   = att_PID(3);

u_posZ = posZ_PID;

Ixx = MoI(1,1);
Iyy = MoI(2,2);
Izz = MoI(3,3);

g = -gvec(3);

phi     = attitude(1); 
theta   = attitude(2);
psi     = attitude(3);


gamma1 = m*(g - u_posZ)/(4*k*cos(theta)*cos(phi)) - (2*b*u_phi*Ixx + u_psi*Izz*k*L)/(4*b*k*L);
gamma2 = m*(g - u_posZ)/(4*k*cos(theta)*cos(phi)) + u_psi*Izz/4/b - u_theta*Iyy/2/k/L;
gamma3 = m*(g - u_posZ)/(4*k*cos(theta)*cos(phi)) - (-2*b*u_phi*Ixx + u_psi*Izz*k*L)/(4*b*k*L);
gamma4 = m*(g - u_posZ)/(4*k*cos(theta)*cos(phi)) + u_psi*Izz/4/b + u_theta*Iyy/2/k/L;


gamma = [gamma1, gamma2, gamma3, gamma4]';

== matlab function My_Nonlinear_with_controller_draft/Altitude Controller1/controller output to torque ==
  data: u input; torque output; MoI input; m input; g input; Theta input
function torque = fcn(u, MoI, m, g, Theta)

u_phi = u(1);
u_theta = u(2);
u_psi = u(3);
F_cz = -u(4);

Ixx = MoI(1,1);
Iyy = MoI(2,2);
Izz = MoI(3,3);

phi = Theta(1);
theta = Theta(2);

torque = [  -Ixx * u_phi;
            -Iyy * u_theta;
            -Izz * u_psi;
            (m * g + m * F_cz)/(k * cos(phi) * cos(theta))];

== matlab function My_Nonlinear_with_controller_draft/Motor Controller1/MATLAB Function ==
  data: L input; gamma output; k input; b input; torque input
function gamma = fcn(L, k, b, torque)
M = [   L*k 0 -L*k 0;
        0, L*k, 0 -L*k;
        b, -b, b, -b;
        1 1 1 1];
M_inv = pinv(M);

gamma = M_inv *torque;
